simulink model "PID"  (R2021a)
settings: Solver=VariableStepAuto  StartTime=0.0  StopTime=10.0  RelTol=1e-3
settings Model: Creator=thibaut  LastModifiedBy=thibaut

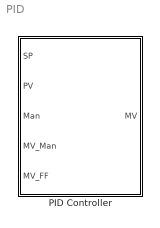
== system PID ==
  PID Controller : Subsystem  mask{T_S=0, MV_Min=0, MV_Max=0, K_C=0, T_I=0, T_D=0, alph=0}
      mask prompts: T_S "Sampling Time [s]"; MV_Min "MV minimum"; MV_Max "MV maximum"; K_C "Control Gain"; T_I "Integrator Time Constant [s]"; T_D "Derivative Time Constant [s]"; alph "Alpha Constant"

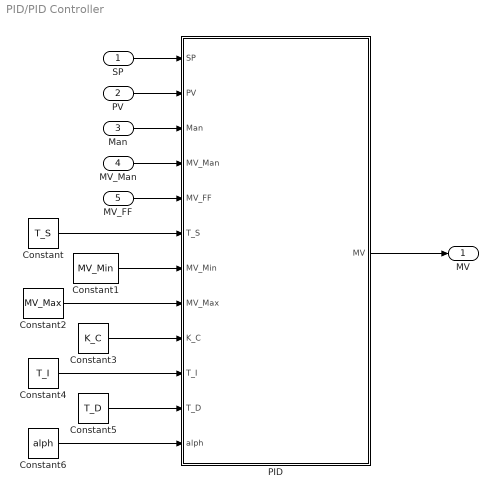
== system PID/PID Controller ==
  SP : Inport
  PV : Inport  Port=2
  Man : Inport  Port=3
  MV_Man : Inport  Port=4
  MV_FF : Inport  Port=5
  Constant : Constant  Value=T_S
  Constant1 : Constant  Value=MV_Min
  Constant2 : Constant  Value=MV_Max
  Constant3 : Constant  Value=K_C
  Constant4 : Constant  Value=T_I
  Constant5 : Constant  Value=T_D
  Constant6 : Constant  Value=alph
  PID : MATLAB Function  TreatAsAtomicUnit=on
  MV : Outport
  wires:
  Constant3/1 -> PID/9(K_C)
  SP/1 -> PID/1(SP)
  PID/1(MV) -> MV/1
  Man/1 -> PID/3(Man)
  MV_FF/1 -> PID/5(MV_FF)
  Constant6/1 -> PID/12(alph)
  Constant2/1 -> PID/8(MV_Max)
  Constant/1 -> PID/6(T_S)
  Constant5/1 -> PID/11(T_D)
  Constant1/1 -> PID/7(MV_Min)
  Constant4/1 -> PID/10(T_I)
  PV/1 -> PID/2(PV)
  MV_Man/1 -> PID/4(MV_Man)

== matlab function PID/PID Controller/PID ==
  data: SP input; MV output; PV input; Man input; MV_Man input; MV_FF input; T_S input; MV_Min input; MV_Max input; K_C input; T_I input; T_D input; alph input
function MV = PID(SP, PV, Man, MV_Man, MV_FF, T_S, MV_Min, MV_Max, K_C, T_I, T_D, alph)
    persistent E_bef
    persistent MVi_bef
    persistent MVd_bef
    
    if isempty(E_bef)
        E_bef = O*SP;
    end
    
    if isempty(MVi_bef)
        MVi_bef = O*SP;
    end
    
    if isempty(MVd_bef)
        MVd_bef = O*SP;
    end

    E = SP-PV;
    T_FD = alph*T_D;
    MVp = K_C*E;
    MVi = MVi_bef + ((K_C*T_S)/T_I)*E;
    MVd = (T_FD/(T_FD+T_S))*MVd_bef + ((K_C*T_D)/(T_FD+T_S))*(E-E_bef);   
    
    if Man == 1 
        MVi = MV_Man - MVp;
    end
    
    if (MVp + MVi) > MV_Max
        MVi = MV_Max - MVp;
    elseif (MVp + MVi) < MV_Min
        MVi = MV_Min - MVp;
    end
    
    MV_FB = MVp + MVi + MVd;
    MV = MV_FB + MV_FF;
    E_bef = E;
    MVi_bef = MVi;
    MVd_bef = MVd;
